simulink model "Upper_Triangular_Example1"  (R2014b)
settings: Solver=ode3  StartTime=0.0  StopTime=100  FixedStep=0.005  RelTol=1e-3
undefined symbols (not defined in the file): v1, v10, v11, v12, v13, v14, v2, v3, v4, v5, v6, v7, v8, v9
settings Model: Creator=QiuJiongzhi  LastModifiedBy=Administrator

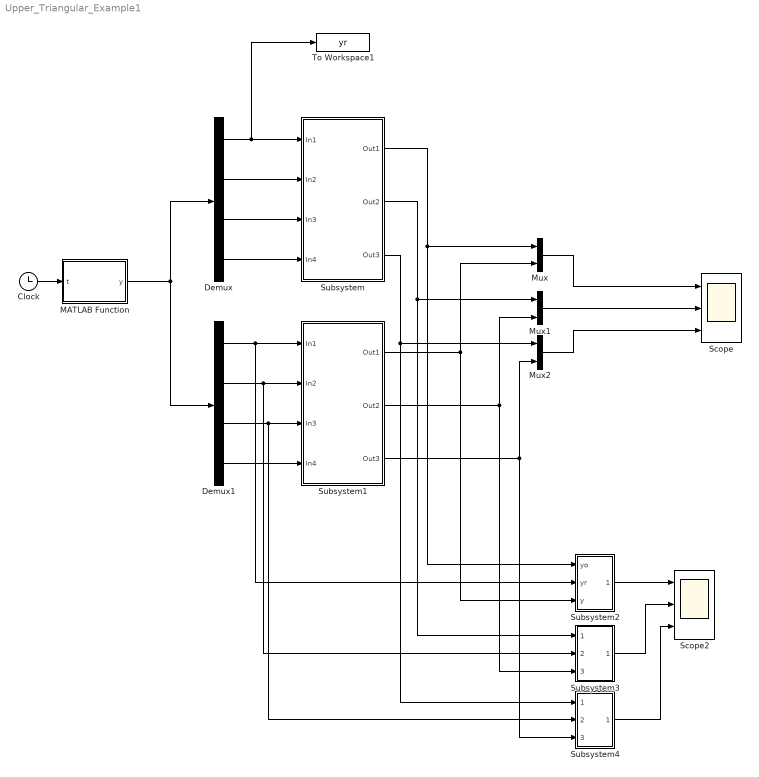
== system Upper_Triangular_Example1 ==
  Clock : Clock
  Demux : Demux
  Demux1 : Demux
  MATLAB Function : MATLAB Function  TreatAsAtomicUnit=on
  Mux : Mux  Inputs=2
  Mux1 : Mux  Inputs=2
  Mux2 : Mux  Inputs=2
  Scope : Scope  NumInputPorts=3
      settings: ShowLegends=on  YMin=-40~-10~-5  YMax=40~30~15
  Scope2 : Scope  NumInputPorts=3
      settings: ShowLegends=on  YMin=-40~-10~-5  YMax=40~30~15  SaveName=ScopeData3
  Subsystem : Subsystem  mask{k1=v1, k2=v2, k3=v3, h1=v4, h2=v5, h3=v6, q1=v7, q2=v8, q3=v9, Center=[10;10;1;1], sigma=1, L=v10, miu1=v11, miu2=v12, phi0=v13, phi1=v14}
  Subsystem1 : Subsystem  mask{k1=v1, k2=v2, k3=v3, h1=v4, h2=v5, h3=v6, q1=v7, q2=v8, q3=v9, Center=[2;2;1;1], sigma=1, L=v10, miu=0, phi0=0, phi1=0}
  Subsystem2 : Subsystem
  Subsystem3 : Subsystem
  Subsystem4 : Subsystem
  To Workspace1 : ToWorkspace  VariableName=yr  SaveFormat=Structure With Time  SampleTime=-1
  wires:
  Subsystem/1(Out1) -> Subsystem2/1(yo), Mux/1
  Subsystem/2(Out2) -> Subsystem3/1(In1), Mux1/1
  Mux/1 -> Scope/1
  Mux1/1 -> Scope/2
  Mux2/1 -> Scope/3
  Subsystem1/1(Out1) -> Subsystem2/3(y), Mux/2
  Subsystem1/2(Out2) -> Mux1/2, Subsystem3/3(In3)
  Subsystem/3(Out3) -> Subsystem4/1(In1), Mux2/1
  Subsystem1/3(Out3) -> Mux2/2, Subsystem4/3(In3)
  Clock/1 -> MATLAB Function/1(t)
  MATLAB Function/1(y) -> Demux/1, Demux1/1
  Demux/1 -> To Workspace1/1, Subsystem/1(In1)
  Demux/2 -> Subsystem/2(In2)
  Demux/3 -> Subsystem/3(In3)
  Demux/4 -> Subsystem/4(In4)
  Demux1/1 -> Subsystem2/2(yr), Subsystem1/1(In1)
  Demux1/2 -> Subsystem3/2(In2), Subsystem1/2(In2)
  Demux1/3 -> Subsystem4/2(In2), Subsystem1/3(In3)
  Demux1/4 -> Subsystem1/4(In4)
  Subsystem2/1(Out1) -> Scope2/1
  Subsystem3/1(Out1) -> Scope2/2
  Subsystem4/1(Out1) -> Scope2/3

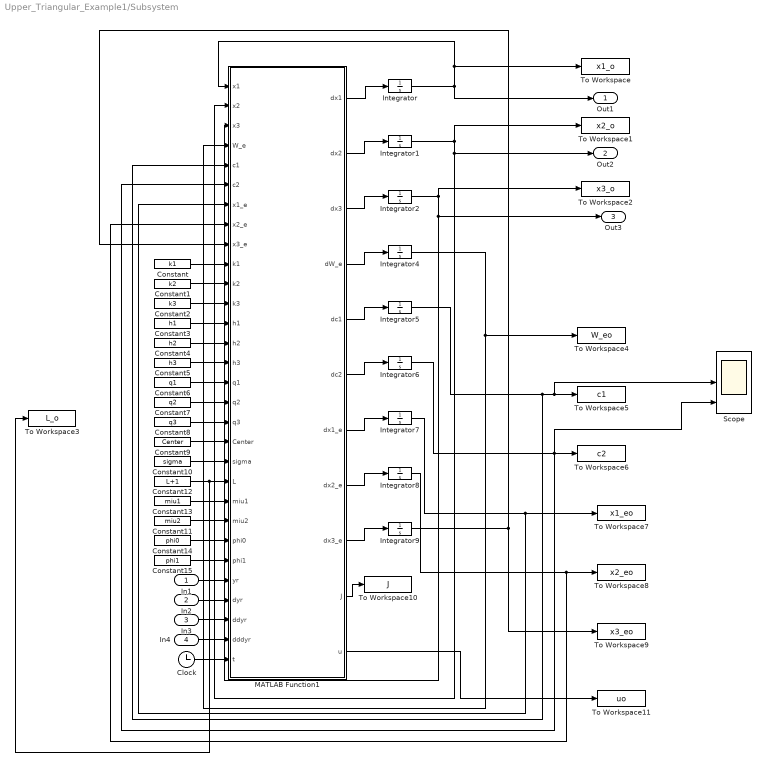
== system Upper_Triangular_Example1/Subsystem ==
  In1 : Inport
  In2 : Inport  Port=2
  In3 : Inport  Port=3
  In4 : Inport  Port=4
  Clock : Clock
  Constant : Constant  Value=k1
  Constant1 : Constant  Value=k2
  Constant10 : Constant  Value=sigma
  Constant11 : Constant  Value=miu2
  Constant12 : Constant  Value=L+1
  Constant13 : Constant  Value=miu1
  Constant14 : Constant  Value=phi0
  Constant15 : Constant  Value=phi1
  Constant2 : Constant  Value=k3
  Constant3 : Constant  Value=h1
  Constant4 : Constant  Value=h2
  Constant5 : Constant  Value=h3
  Constant6 : Constant  Value=q1
  Constant7 : Constant  Value=q2
  Constant8 : Constant  Value=q3
  Constant9 : Constant  Value=Center
  Integrator : Integrator  InitialCondition=20
  Integrator1 : Integrator  InitialCondition=-0.5
  Integrator2 : Integrator  InitialCondition=0.5
  Integrator4 : Integrator  InitialCondition=[0;0;0;0;0]
  Integrator{5..9} (5 alike) : Integrator
  MATLAB Function1 : MATLAB Function  TreatAsAtomicUnit=on
  Scope : Scope  NumInputPorts=3
      settings: ShowLegends=on  YMin=-5~-5~-5  YMax=5~5~5
  To Workspace : ToWorkspace  VariableName=x1_o  SaveFormat=Structure With Time  SampleTime=-1
  To Workspace1 : ToWorkspace  VariableName=x2_o  SaveFormat=Structure With Time  SampleTime=-1
  To Workspace10 : ToWorkspace  VariableName=J  SaveFormat=Structure With Time  SampleTime=-1
  To Workspace11 : ToWorkspace  VariableName=uo  SaveFormat=Structure With Time  SampleTime=-1
  To Workspace2 : ToWorkspace  VariableName=x3_o  SaveFormat=Structure With Time  SampleTime=-1
  To Workspace3 : ToWorkspace  VariableName=L_o  SaveFormat=Structure With Time  SampleTime=-1
  To Workspace4 : ToWorkspace  VariableName=W_eo  SaveFormat=Structure With Time  SampleTime=-1
  To Workspace5 : ToWorkspace  VariableName=c1  SaveFormat=Structure With Time  SampleTime=-1
  To Workspace6 : ToWorkspace  VariableName=c2  SaveFormat=Structure With Time  SampleTime=-1
  To Workspace7 : ToWorkspace  VariableName=x1_eo  SaveFormat=Structure With Time  SampleTime=-1
  To Workspace8 : ToWorkspace  VariableName=x2_eo  SaveFormat=Structure With Time  SampleTime=-1
  To Workspace9 : ToWorkspace  VariableName=x3_eo  SaveFormat=Structure With Time  SampleTime=-1
  Out1 : Outport
  Out2 : Outport  Port=2
  Out3 : Outport  Port=3
  wires:
  MATLAB Function1/1(dx1) -> Integrator/1
  Integrator2/1 -> To Workspace2/1, MATLAB Function1/3(x3), Out3/1
  Integrator7/1 -> MATLAB Function1/7(x1_e), To Workspace7/1
  Integrator6/1 -> Scope/3, MATLAB Function1/6(c2), To Workspace6/1
  Integrator4/1 -> MATLAB Function1/4(W_e), To Workspace4/1
  Integrator5/1 -> MATLAB Function1/5(c1), Scope/2, To Workspace5/1
  Integrator9/1 -> To Workspace9/1, MATLAB Function1/9(x3_e)
  Integrator8/1 -> MATLAB Function1/8(x2_e), To Workspace8/1
  Integrator/1 -> MATLAB Function1/1(x1), To Workspace/1, Out1/1
  Integrator1/1 -> To Workspace1/1, MATLAB Function1/2(x2), Out2/1
  MATLAB Function1/10(J) -> To Workspace10/1
  In1/1 -> MATLAB Function1/26(yr)
  In2/1 -> MATLAB Function1/27(dyr)
  In3/1 -> MATLAB Function1/28(ddyr)
  In4/1 -> MATLAB Function1/29(dddyr)
  MATLAB Function1/2(dx2) -> Integrator1/1
  MATLAB Function1/3(dx3) -> Integrator2/1
  MATLAB Function1/4(dW_e) -> Integrator4/1
  MATLAB Function1/5(dc1) -> Integrator5/1
  MATLAB Function1/6(dc2) -> Integrator6/1
  MATLAB Function1/7(dx1_e) -> Integrator7/1
  MATLAB Function1/8(dx2_e) -> Integrator8/1
  MATLAB Function1/9(dx3_e) -> Integrator9/1
  MATLAB Function1/11(u) -> To Workspace11/1
  Constant14/1 -> MATLAB Function1/24(phi0)
  Constant15/1 -> MATLAB Function1/25(phi1)
  Constant13/1 -> MATLAB Function1/22(miu1)
  Constant12/1 -> To Workspace3/1, MATLAB Function1/21(L)
  Constant10/1 -> MATLAB Function1/20(sigma)
  Constant9/1 -> MATLAB Function1/19(Center)
  Constant8/1 -> MATLAB Function1/18(q3)
  Constant7/1 -> MATLAB Function1/17(q2)
  Constant6/1 -> MATLAB Function1/16(q1)
  Constant5/1 -> MATLAB Function1/15(h3)
  Constant4/1 -> MATLAB Function1/14(h2)
  Constant3/1 -> MATLAB Function1/13(h1)
  Constant2/1 -> MATLAB Function1/12(k3)
  Constant1/1 -> MATLAB Function1/11(k2)
  Constant/1 -> MATLAB Function1/10(k1)
  Clock/1 -> MATLAB Function1/30(t)
  Constant11/1 -> MATLAB Function1/23(miu2)

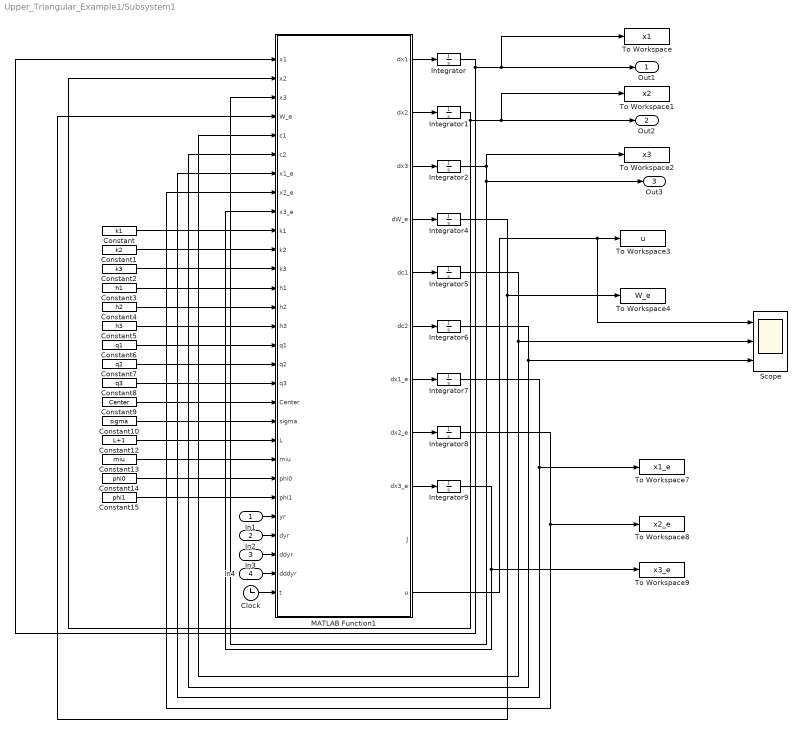
== system Upper_Triangular_Example1/Subsystem1 ==
  In1 : Inport
  In2 : Inport  Port=2
  In3 : Inport  Port=3
  In4 : Inport  Port=4
  Clock : Clock
  Constant : Constant  Value=k1
  Constant1 : Constant  Value=k2
  Constant10 : Constant  Value=sigma
  Constant12 : Constant  Value=L+1
  Constant13 : Constant  Value=miu
  Constant14 : Constant  Value=phi0
  Constant15 : Constant  Value=phi1
  Constant2 : Constant  Value=k3
  Constant3 : Constant  Value=h1
  Constant4 : Constant  Value=h2
  Constant5 : Constant  Value=h3
  Constant6 : Constant  Value=q1
  Constant7 : Constant  Value=q2
  Constant8 : Constant  Value=q3
  Constant9 : Constant  Value=Center
  Integrator : Integrator  InitialCondition=20
  Integrator1 : Integrator  InitialCondition=-0.5
  Integrator2 : Integrator  InitialCondition=0.5
  Integrator4 : Integrator  InitialCondition=[0;0;0;0;0]
  Integrator{5..9} (5 alike) : Integrator
  MATLAB Function1 : MATLAB Function  TreatAsAtomicUnit=on
  Scope : Scope  NumInputPorts=3
      settings: ShowLegends=on  YMin=-5~-5~-5  YMax=5~5~5
  To Workspace : ToWorkspace  VariableName=x1  SaveFormat=Structure With Time  SampleTime=-1
  To Workspace1 : ToWorkspace  VariableName=x2  SaveFormat=Structure With Time  SampleTime=-1
  To Workspace2 : ToWorkspace  VariableName=x3  SaveFormat=Structure With Time  SampleTime=-1
  To Workspace3 : ToWorkspace  VariableName=u  SaveFormat=Structure With Time  SampleTime=-1
  To Workspace4 : ToWorkspace  VariableName=W_e  SaveFormat=Structure With Time  SampleTime=-1
  To Workspace7 : ToWorkspace  VariableName=x1_e  SaveFormat=Structure With Time  SampleTime=-1
  To Workspace8 : ToWorkspace  VariableName=x2_e  SaveFormat=Structure With Time  SampleTime=-1
  To Workspace9 : ToWorkspace  VariableName=x3_e  SaveFormat=Structure With Time  SampleTime=-1
  Out1 : Outport
  Out2 : Outport  Port=2
  Out3 : Outport  Port=3
  wires:
  MATLAB Function1/3(dx3) -> Integrator2/1
  MATLAB Function1/2(dx2) -> Integrator1/1
  Constant14/1 -> MATLAB Function1/23(phi0)
  MATLAB Function1/1(dx1) -> Integrator/1
  Constant/1 -> MATLAB Function1/10(k1)
  Constant3/1 -> MATLAB Function1/13(h1)
  Constant9/1 -> MATLAB Function1/19(Center)
  Integrator2/1 -> Out3/1, MATLAB Function1/3(x3), To Workspace2/1
  Integrator7/1 -> To Workspace7/1, MATLAB Function1/7(x1_e)
  MATLAB Function1/7(dx1_e) -> Integrator7/1
  MATLAB Function1/9(dx3_e) -> Integrator9/1
  Constant2/1 -> MATLAB Function1/12(k3)
  Integrator6/1 -> Scope/3, MATLAB Function1/6(c2)
  Constant10/1 -> MATLAB Function1/20(sigma)
  Constant15/1 -> MATLAB Function1/24(phi1)
  MATLAB Function1/11(u) -> Scope/1, To Workspace3/1
  Integrator4/1 -> To Workspace4/1, MATLAB Function1/4(W_e)
  MATLAB Function1/5(dc1) -> Integrator5/1
  Constant12/1 -> MATLAB Function1/21(L)
  Constant5/1 -> MATLAB Function1/15(h3)
  Constant7/1 -> MATLAB Function1/17(q2)
  Constant8/1 -> MATLAB Function1/18(q3)
  Constant6/1 -> MATLAB Function1/16(q1)
  Constant4/1 -> MATLAB Function1/14(h2)
  Integrator5/1 -> MATLAB Function1/5(c1), Scope/2
  MATLAB Function1/8(dx2_e) -> Integrator8/1
  MATLAB Function1/4(dW_e) -> Integrator4/1
  Constant1/1 -> MATLAB Function1/11(k2)
  Integrator9/1 -> MATLAB Function1/9(x3_e), To Workspace9/1
  Constant13/1 -> MATLAB Function1/22(miu)
  Integrator8/1 -> To Workspace8/1, MATLAB Function1/8(x2_e)
  In2/1 -> MATLAB Function1/26(dyr)
  In3/1 -> MATLAB Function1/27(ddyr)
  In4/1 -> MATLAB Function1/28(dddyr)
  In1/1 -> MATLAB Function1/25(yr)
  Integrator/1 -> To Workspace/1, Out1/1, MATLAB Function1/1(x1)
  MATLAB Function1/6(dc2) -> Integrator6/1
  Integrator1/1 -> MATLAB Function1/2(x2), To Workspace1/1, Out2/1
  Clock/1 -> MATLAB Function1/29(t)

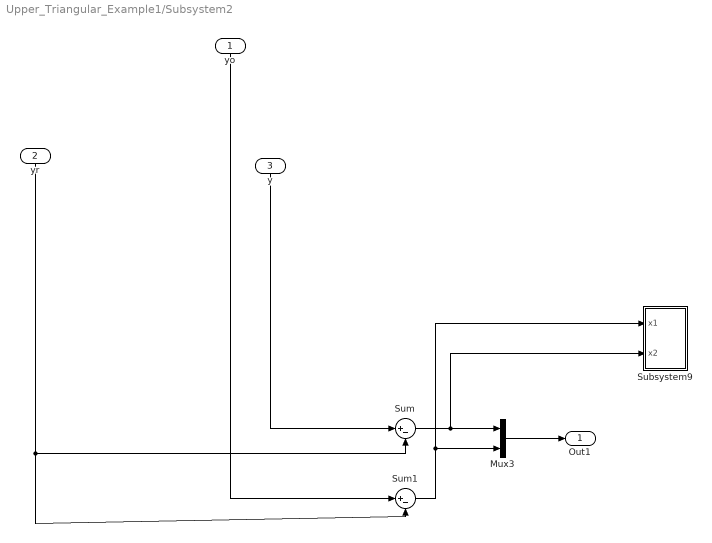
== system Upper_Triangular_Example1/Subsystem2 ==
  yo : Inport
  yr : Inport  Port=2
  y : Inport  Port=3
  Mux3 : Mux  Inputs=2
  Subsystem9 : Subsystem
  Sum : Sum  Inputs=|+-
  Sum1 : Sum  Inputs=|+-
  Out1 : Outport
  wires:
  yo/1 -> Sum1/1
  yr/1 -> Sum/2, Sum1/2
  y/1 -> Sum/1
  Mux3/1 -> Out1/1
  Sum1/1 -> Subsystem9/1(x1), Mux3/2
  Sum/1 -> Subsystem9/2(x2), Mux3/1

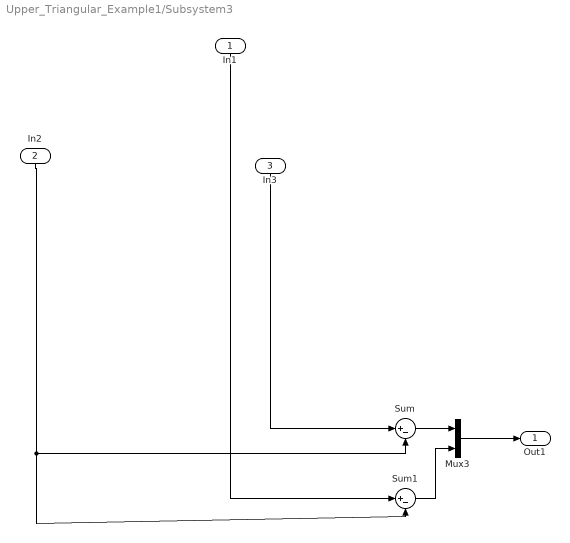
== system Upper_Triangular_Example1/Subsystem3 ==
  In1 : Inport
  In2 : Inport  Port=2
  In3 : Inport  Port=3
  Mux3 : Mux  Inputs=2
  Sum : Sum  Inputs=|+-
  Sum1 : Sum  Inputs=|+-
  Out1 : Outport
  wires:
  In1/1 -> Sum1/1
  In2/1 -> Sum/2, Sum1/2
  In3/1 -> Sum/1
  Mux3/1 -> Out1/1
  Sum/1 -> Mux3/1
  Sum1/1 -> Mux3/2

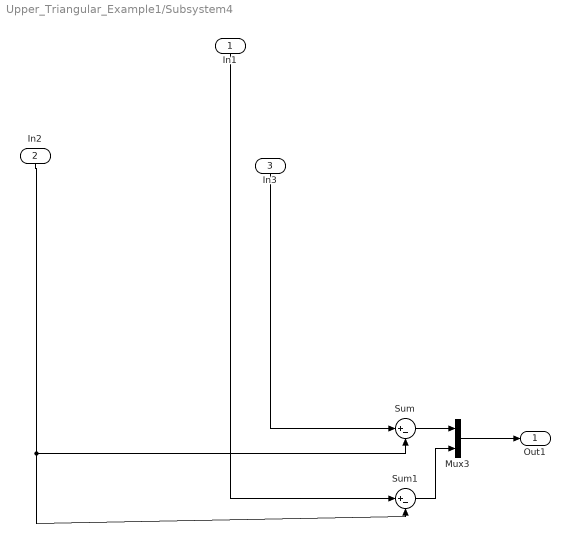
== system Upper_Triangular_Example1/Subsystem4 ==
  In1 : Inport
  In2 : Inport  Port=2
  In3 : Inport  Port=3
  Mux3 : Mux  Inputs=2
  Sum : Sum  Inputs=|+-
  Sum1 : Sum  Inputs=|+-
  Out1 : Outport
  wires:
  In1/1 -> Sum1/1
  In2/1 -> Sum/2, Sum1/2
  In3/1 -> Sum/1
  Mux3/1 -> Out1/1
  Sum/1 -> Mux3/1
  Sum1/1 -> Mux3/2

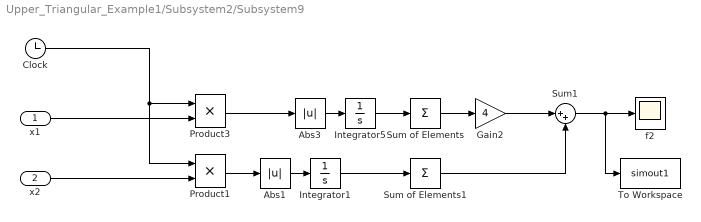
== system Upper_Triangular_Example1/Subsystem2/Subsystem9 ==
  x1 : Inport
  x2 : Inport  Port=2
  Abs1 : Abs
  Abs3 : Abs
  Clock : Clock
  Gain2 : Gain  Gain=4
  Integrator1 : Integrator
  Integrator5 : Integrator
  Product1 : Product
  Product3 : Product
  Sum of Elements : Sum  Inputs=+
  Sum of Elements1 : Sum  Inputs=+
  Sum1 : Sum  Inputs=|++
  To Workspace : ToWorkspace  VariableName=simout1  SaveFormat=Structure With Time  SampleTime=-1
  f2 : Scope
      settings: TimeRange=24.44047636723186  YMin=-2  YMax=3  SaveName=f2
  wires:
  Clock/1 -> Product1/1, Product3/1
  Abs3/1 -> Integrator5/1
  x1/1 -> Product3/2
  Sum1/1 -> To Workspace/1, f2/1
  x2/1 -> Product1/2
  Product1/1 -> Abs1/1
  Abs1/1 -> Integrator1/1
  Integrator1/1 -> Sum of Elements1/1
  Sum of Elements/1 -> Gain2/1
  Sum of Elements1/1 -> Sum1/2
  Integrator5/1 -> Sum of Elements/1
  Product3/1 -> Abs3/1
  Gain2/1 -> Sum1/1

== matlab function Upper_Triangular_Example1/Subsystem1/MATLAB Function1 ==
  data: dx1 output; dx2 output; dx3 output; dW_e output; dc1 output; dc2 output; dx1_e output; dx2_e output; dx3_e output; x1 input; J output; x2 input; x3 input; W_e input; c1 input; c2 input; x1_e input; x2_e input; x3_e input; k1 input; k2 input; k3 input; h1 input; h2 input; h3 input; q1 input; q2 input; q3 input; Center input; sigma input; L input; miu input; phi0 input; phi1 input; yr input; dyr input; ddyr input; dddyr input; u output; t input
function [dx1,dx2,dx3,dW_e,dc1,dc2,dx1_e,dx2_e,dx3_e,J,u] = fcn(x1,x2,x3,W_e,c1,c2,x1_e,x2_e,x3_e,k1,k2,k3,h1,h2,h3,q1,q2,q3,Center,sigma,L,miu,phi0,phi1,yr,dyr,ddyr,dddyr,t)
%#codegen
y = x1;
J = miu*(L^(-3)*(x1_e - yr))^2 + miu*(L^(-3)*(x1_e - y))^2;
dc1 = -2*miu*(L^(-3)*(x1_e - yr));
dc2 = -2*miu*(L^(-3)*(y - x1_e));

z1 = L^(-3)*(x1_e - yr) - c1;
z2 = L^(-2)*(x2_e - dyr);z3 = L^(-1)*(x3_e - ddyr);
zeta_h = h1*z1 + h2*z2 + h3*z3;
zeta_qn = q1*z1 + q2*z2 + q3*z3;

base = [-2,-1,0,1,2];
co = [Center(1,1).*base;Center(2,1).*base;Center(3,1).*base;Center(4,1).*base];
co1 = co(:,1);co2 = co(:,2);co3 = co(:,3);co4 = co(:,4);co5 = co(:,5);
x = [y;x1_e;x2_e;x3_e];

Xi = [exp(-(norm(x-co1,2))^2/(2*sigma^2));
    exp(-(norm(x-co2,2))^2/(2*sigma^2));
    exp(-(norm(x-co3,2))^2/(2*sigma^2));
    exp(-(norm(x-co4,2))^2/(2*sigma^2));
    exp(-(norm(x-co5,2))^2/(2*sigma^2))];
Pi = 1;

dW_e = Pi*Xi*zeta_qn - phi1*Pi*W_e;


u = dddyr - zeta_h;
%rou = abs(u);
%dL = max(varpi^(-1)*L*(L^(-2)*rou^2 - k_U*L^(-1)),0);
dx1_e = x2_e + k1*L^(-1)*(y - x1_e) - L^(3)*dc2 - k1*L^(2)*c2;
dx2_e = x3_e + k2*L^(-2)*(y - x1_e) - (k2)*L^(2)*c2;
dx3_e = u + k3*L^(-3)*(y - x1_e) - (k3)*L^(2)*c2;
%% System
dx1 = x2 + 0.1*sin(x2)*tanh(u)*x3;
dx2 = x3;
dx3 = u;

== matlab function Upper_Triangular_Example1/MATLAB Function ==
  data: t input; y output
function y = fcn(t)
%#codegen

y = [1*sin(t);
    1*cos(t);
    -1*sin(t);
    -1*cos(t)];

== matlab function Upper_Triangular_Example1/Subsystem/MATLAB Function1 ==
  data: x1 input; x2 input; x3 input; W_e input; c1 input; c2 input; x1_e input; x2_e input; x3_e input; k1 input; k2 input; k3 input; h1 input; h2 input; h3 input; q1 input; q2 input; q3 input; Center input; sigma input; L input; miu1 input; miu2 input; phi0 input; phi1 input; yr input; dyr input; ddyr input; dddyr input; dx1 output; dx2 output; dx3 output; dW_e output; dc1 output; dc2 output; dx1_e output; dx2_e output; dx3_e output; J output; u output; t input
function [dx1,dx2,dx3,dW_e,dc1,dc2,dx1_e,dx2_e,dx3_e,J,u] = fcn(x1,x2,x3,W_e,c1,c2,x1_e,x2_e,x3_e,k1,k2,k3,h1,h2,h3,q1,q2,q3,Center,sigma,L,miu1,miu2,phi0,phi1,yr,dyr,ddyr,dddyr,t)
%#codegen
y = x1;
J = miu1*(L^(-3)*(x1_e - yr))^2 + miu2*(L^(-3)*(x1_e - y))^2;
dc1 = -2*miu1*(L^(-3)*(x1_e - yr));
dc2 = -2*miu2*(L^(-3)*(y - x1_e));

z1 = L^(-3)*(x1_e - yr) - c1;
z2 = L^(-2)*(x2_e - dyr);z3 = L^(-1)*(x3_e - ddyr);
zeta_h = h1*z1 + h2*z2 + h3*z3;
zeta_qn = q1*z1 + q2*z2 + q3*z3;

base = [-2,-1,0,1,2];
co = [Center(1,1).*base;Center(2,1).*base;Center(3,1).*base;Center(4,1).*base];
co1 = co(:,1);co2 = co(:,2);co3 = co(:,3);co4 = co(:,4);co5 = co(:,5);
x = [y;x1_e;x2_e;x3_e];

Xi = [exp(-(norm(x-co1,2))^2/(2*sigma^2));
    exp(-(norm(x-co2,2))^2/(2*sigma^2));
    exp(-(norm(x-co3,2))^2/(2*sigma^2));
    exp(-(norm(x-co4,2))^2/(2*sigma^2));
    exp(-(norm(x-co5,2))^2/(2*sigma^2))];
Pi = 1;

dW_e = Pi*Xi*zeta_qn - phi1*Pi*W_e;


u = dddyr - zeta_h - L*(W_e'*Xi + 0.5*phi0*zeta_qn);
%rou = abs(u);
%dL = max(varpi^(-1)*L*(L^(-2)*rou^2 - k_U*L^(-1)),0);
dx1_e = x2_e + k1*L^(-1)*(y - x1_e) - L^(3)*dc2 - k1*L^(2)*c2;
dx2_e = x3_e + k2*L^(-2)*(y - x1_e) - (k2)*L^(2)*c2;
dx3_e = u + k3*L^(-3)*(y - x1_e) - (k3)*L^(2)*c2;
%% System
dx1 = x2 + 0.1*sin(x2)*tanh(u)*x3;
dx2 = x3;
dx3 = u;
